simulink model "RobotArmControl"  (R2014a)
settings: Solver=ode45  StartTime=0.0  StopTime=10  RelTol=1e-3
values from neighbouring files (symbols this model uses):
  a1 = 0    [MainRobotControl.m]    (also in RobotParameters.m; Trajectory_PlanningRot.m; Trajectory_planning.m = x0; taskspace_v1.m = 5.66666666667)
  a2 = 0.2    [MainRobotControl.m]    (also in RobotParameters.m; Trajectory_PlanningRot.m = 0; Trajectory_planning.m = xdot0; taskspace_v1.m = 20)
  a3 = 0.2    [MainRobotControl.m]    (also in RobotParameters.m; Trajectory_PlanningRot.m = (3*h - (2*thetadot_0 + thetadot_f)*T)/(T*T); Trajectory_planning.m = (3*h - (2*xdot0 + xdotf)*T)/(T*T); taskspace_v1.m = 26.8333333333)
  d1 = 0.2    [MainRobotControl.m]    (also in RobotParameters.m; taskspace_v1.m = 15.8333333333)
  d5 = 0.07    [MainRobotControl.m]    (also in RobotParameters.m; taskspace_v1.m = 10)
  gear_eff = 0.85    [RobotParameters.m]
  kphi = 37.83e-3    (= 0.03783)    [RobotParameters.m]
  Kv = 4.09e-4    (= 0.000409)    [RobotParameters.m]
  Ra = 5.84    [RobotParameters.m]
  ratio = 19    [RobotParameters.m]
  tau_e = La/Ra    (= 9.58904109589e-05)    [RobotParameters.m]
  tau_m = Jrob/Kv    (= 8.25476772616)    [RobotParameters.m]
libraries: simulink x6
settings Model: Creator=Guillaume  LastModifiedBy=Guillaume

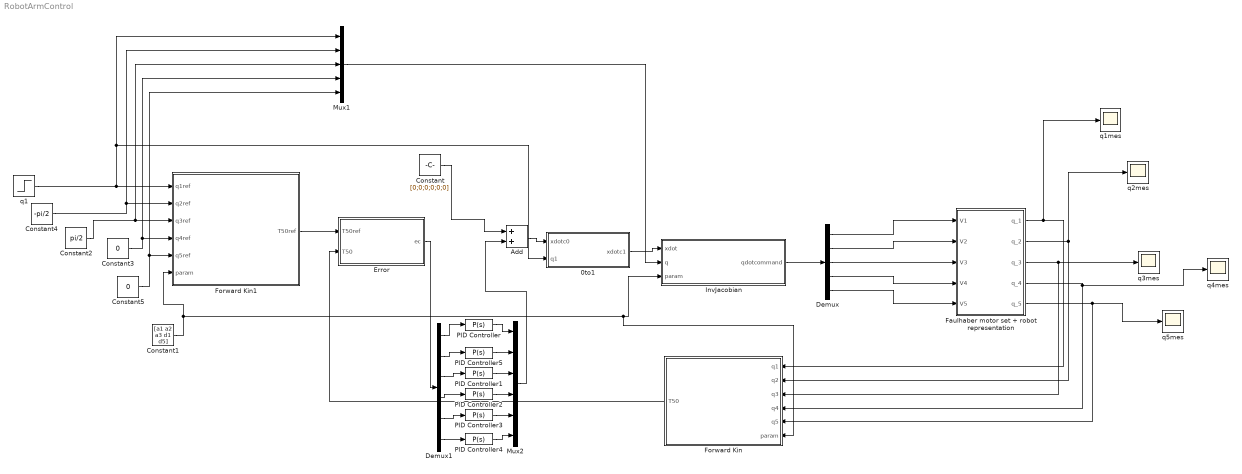
== system RobotArmControl ==
  0to1 : MATLAB Function  TreatAsAtomicUnit=on
  Add : Sum
  Constant : Constant  Value=[0;0;0;0;0;0]
  Constant1 : Constant  Value=[a1 a2 a3 d1 d5]
  Constant2 : Constant  Value=pi/2
  Constant3 : Constant  Value=0
  Constant4 : Constant  Value=-pi/2
  Constant5 : Constant  Value=0
  Demux : Demux  Outputs=5
  Demux1 : Demux  Outputs=6
  Error : MATLAB Function  TreatAsAtomicUnit=on
  Faulhaber motor set + robot representation : Subsystem
  Forward Kin : MATLAB Function  TreatAsAtomicUnit=on
  Forward Kin1 : MATLAB Function  TreatAsAtomicUnit=on
  InvJacobian : MATLAB Function  TreatAsAtomicUnit=on
  Mux1 : Mux  Inputs=5
  Mux2 : Mux  Inputs=6
  PID Controller{,1..5} (6 alike) : simulink/Continuous/PID Controller  Controller=P  TimeDomain=Continuous-time  SampleTime=1  IntegratorMethod=Forward Euler  FilterMethod=Forward Euler  Form=Parallel  P=1e-5  I=1  D=0  N=100  InitialConditionSource=internal  InitialConditionForIntegrator=0  InitialConditionForFilter=0  ExternalReset=none  LimitOutput=off  UpperSaturationLimit=inf  LowerSaturationLimit=-inf  LinearizeAsGain=on  AntiWindupMode=none  Kb=1  TrackingMode=off  Kt=1  PParamMin=[]  PParamMax=[]  IParamMin=[]  IParamMax=[]  DParamMin=[]  DParamMax=[]  NParamMin=[]  NParamMax=[]  KbParamMin=[]  KbParamMax=[]  KtParamMin=[]  KtParamMax=[]  POutMin=[]  POutMax=[]  IOutMin=[]  IOutMax=[]  DOutMin=[]  DOutMax=[]  NOutMin=[]  NOutMax=[]  KbOutMin=[]  KbOutMax=[]  KtOutMin=[]  KtOutMax=[]  IntegratorOutMin=[]  IntegratorOutMax=[]  FilterOutMin=[]  FilterOutMax=[]  SumOutMin=[]  SumOutMax=[]  SumI1OutMin=[]  SumI1OutMax=[]  SumI2OutMin=[]  SumI2OutMax=[]  SumI3OutMin=[]  SumI3OutMax=[]  SumDOutMin=[]  SumDOutMax=[]  SaturationOutMin=[]  SaturationOutMax=[]  IntegratorContinuousStateAttributes=''  IntegratorStateMustResolveToSignalObject=off  IntegratorRTWStateStorageClass=Auto  FilterContinuousStateAttributes=''  FilterStateMustResolveToSignalObject=off  FilterRTWStateStorageClass=Auto
  q1 : Step  After=pi/20  SampleTime=0
  q1mes : Scope
  q2mes : Scope
  q3mes : Scope
      settings: SaveName=ScopeData2
  q4mes : Scope
      settings: SaveName=ScopeData3
  q5mes : Scope
      settings: SaveName=ScopeData4
  wires:
  Faulhaber motor set + robot representation/1(q_1) -> q1mes/1, Forward Kin/1(q1)
  Faulhaber motor set + robot representation/2(q_2) -> Forward Kin/2(q2), q2mes/1
  Faulhaber motor set + robot representation/3(q_3) -> q3mes/1, Forward Kin/3(q3)
  Faulhaber motor set + robot representation/4(q_4) -> q4mes/1, Forward Kin/4(q4)
  Faulhaber motor set + robot representation/5(q_5) -> q5mes/1, Forward Kin/5(q5)
  InvJacobian/1(qdotcommand) -> Demux/1
  Demux/1 -> Faulhaber motor set + robot representation/1(V1)
  Demux/2 -> Faulhaber motor set + robot representation/2(V2)
  Demux/3 -> Faulhaber motor set + robot representation/3(V3)
  Demux/4 -> Faulhaber motor set + robot representation/4(V4)
  Demux/5 -> Faulhaber motor set + robot representation/5(V5)
  0to1/1(xdotc1) -> InvJacobian/1(xdot)
  Add/1 -> 0to1/1(xdotc0)
  Constant/1 -> Add/1
  Forward Kin/1(T50) -> Error/2(T50)
  Forward Kin1/1(T50ref) -> Error/1(T50ref)
  q1/1 -> 0to1/2(q1), Mux1/1, Forward Kin1/1(q1ref)
  Constant4/1 -> Mux1/2, Forward Kin1/2(q2ref)
  Constant2/1 -> Mux1/3, Forward Kin1/3(q3ref)
  Constant3/1 -> Mux1/4, Forward Kin1/4(q4ref)
  Constant5/1 -> Mux1/5, Forward Kin1/5(q5ref)
  Mux1/1 -> InvJacobian/2(q)
  Constant1/1 -> Forward Kin/6(param), InvJacobian/3(param), Forward Kin1/6(param)
  Error/1(ec) -> Demux1/1
  Demux1/1 -> PID Controller/1
  PID Controller/1 -> Mux2/1
  PID Controller4/1 -> Mux2/6
  Demux1/6 -> PID Controller4/1
  Demux1/5 -> PID Controller3/1
  PID Controller3/1 -> Mux2/5
  Demux1/4 -> PID Controller2/1
  PID Controller2/1 -> Mux2/4
  Demux1/3 -> PID Controller1/1
  PID Controller1/1 -> Mux2/3
  PID Controller5/1 -> Mux2/2
  Demux1/2 -> PID Controller5/1
  Mux2/1 -> Add/2

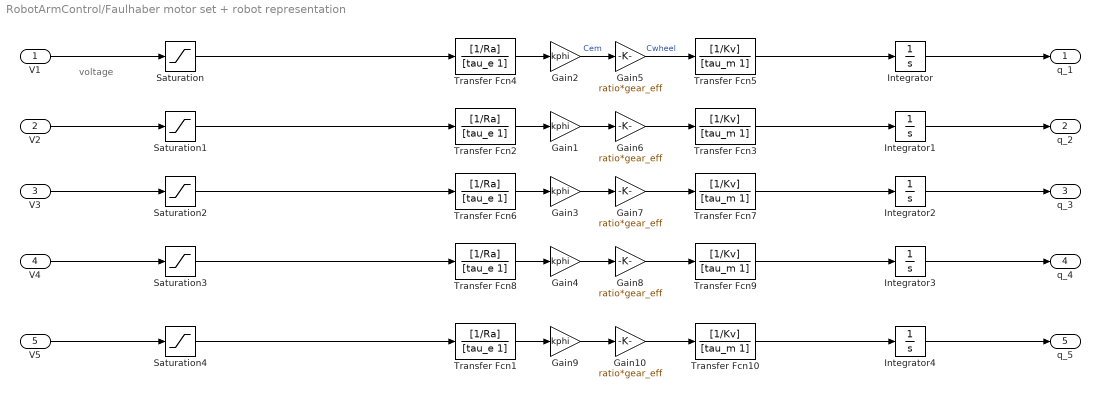
== system RobotArmControl/Faulhaber motor set + robot representation ==
  note: voltage
  V1 : Inport
  V2 : Inport  Port=2
  V3 : Inport  Port=3
  V4 : Inport  Port=4
  V5 : Inport  Port=5
  Gain{1..4,9} (5 alike) : Gain  Gain=kphi
  Gain{5..8,10} (5 alike) : Gain  Gain=ratio*gear_eff
  Integrator{,1..4} (5 alike) : Integrator
  Saturation{,1..4} (5 alike) : Saturate  UpperLimit=52/0.036
  Transfer Fcn{1..2,4,6,8} (5 alike) : TransferFcn  Numerator=[1/Ra]  Denominator=[tau_e 1]
  Transfer Fcn{3,5,7,9..10} (5 alike) : TransferFcn  Numerator=[1/Kv]  Denominator=[tau_m 1]
  q_1 : Outport
  q_2 : Outport  Port=2
  q_3 : Outport  Port=3
  q_4 : Outport  Port=4
  q_5 : Outport  Port=5
  wires:
  Transfer Fcn5/1 -> Integrator/1
  Saturation/1 -> Transfer Fcn4/1
  Transfer Fcn3/1 -> Integrator1/1
  V2/1 -> Saturation1/1
  Saturation1/1 -> Transfer Fcn2/1
  V1/1 -> Saturation/1
  Transfer Fcn7/1 -> Integrator2/1
  V3/1 -> Saturation2/1
  Saturation2/1 -> Transfer Fcn6/1
  Transfer Fcn9/1 -> Integrator3/1
  V4/1 -> Saturation3/1
  Saturation3/1 -> Transfer Fcn8/1
  Transfer Fcn2/1 -> Gain1/1
  Gain1/1 -> Gain6/1
  Transfer Fcn4/1 -> Gain2/1
  Gain2/1 -> Gain5/1  "Cem"
  Transfer Fcn6/1 -> Gain3/1
  Gain3/1 -> Gain7/1
  Transfer Fcn8/1 -> Gain4/1
  Gain4/1 -> Gain8/1
  Gain5/1 -> Transfer Fcn5/1  "Cwheel"
  Gain6/1 -> Transfer Fcn3/1
  Gain7/1 -> Transfer Fcn7/1
  Gain8/1 -> Transfer Fcn9/1
  Integrator/1 -> q_1/1
  Integrator3/1 -> q_4/1
  Integrator2/1 -> q_3/1
  Integrator1/1 -> q_2/1
  Transfer Fcn10/1 -> Integrator4/1
  V5/1 -> Saturation4/1
  Saturation4/1 -> Transfer Fcn1/1
  Transfer Fcn1/1 -> Gain9/1
  Gain9/1 -> Gain10/1
  Gain10/1 -> Transfer Fcn10/1
  Integrator4/1 -> q_5/1

== matlab function RobotArmControl/InvJacobian ==
  data: xdot input; qdotcommand output; q input; param input
function qdotcommand   = InvJacobian5by5(xdot,q,param)
%UNTITLED2 Summary of this function goes here
%   Detailed explanation goes here

%ATTENTION xdot must be expressed in referential 1 !!
%note  : pas de prise en compte d'une commande de omega sur x1.
%supposée zero tout le temps

% invJ5by5 = [                                                                                        0,                                                                                        0,                     1/(a1 + a3*cos(t2 + t3) + a2*cos(t2) - d5*sin(t2 + t3 + t4)),                   0,                                                                                                                                                                                                           0;
%                         -cos(t2 + t3)/(a2*cos(t2 + t3)*sin(t2) - a2*sin(t2 + t3)*cos(t2)),                        -sin(t2 + t3)/(a2*cos(t2 + t3)*sin(t2) - a2*sin(t2 + t3)*cos(t2)),                                                                                0,                   0,                                                                                -(d5*cos(t2 + t3 + t4)*cos(t2 + t3) + d5*sin(t2 + t3 + t4)*sin(t2 + t3))/(a2*cos(t2 + t3)*sin(t2) - a2*sin(t2 + t3)*cos(t2));
%  (a3*cos(t2 + t3) + a2*cos(t2))/(a2*a3*cos(t2 + t3)*sin(t2) - a2*a3*sin(t2 + t3)*cos(t2)), (a3*sin(t2 + t3) + a2*sin(t2))/(a2*a3*cos(t2 + t3)*sin(t2) - a2*a3*sin(t2 + t3)*cos(t2)),                                                                                0,                   0, (a3*d5*sin(t2 + t3 + t4)*sin(t2 + t3) + a2*d5*cos(t2 + t3 + t4)*cos(t2) + a2*d5*sin(t2 + t3 + t4)*sin(t2) + a3*d5*cos(t2 + t3 + t4)*cos(t2 + t3))/(a2*a3*cos(t2 + t3)*sin(t2) - a2*a3*sin(t2 + t3)*cos(t2));
%                              -cos(t2)/(a3*cos(t2 + t3)*sin(t2) - a3*sin(t2 + t3)*cos(t2)),                             -sin(t2)/(a3*cos(t2 + t3)*sin(t2) - a3*sin(t2 + t3)*cos(t2)),                                                                                0,                   0,                                      -(a3*sin(t2 + t3)*cos(t2) - a3*cos(t2 + t3)*sin(t2) + d5*cos(t2 + t3 + t4)*cos(t2) + d5*sin(t2 + t3 + t4)*sin(t2))/(a3*cos(t2 + t3)*sin(t2) - a3*sin(t2 + t3)*cos(t2));
%                                                                                         0,                                                                                        0, 1/(cos(t2 + t3 + t4)*(a1 + a3*cos(t2 + t3) + a2*cos(t2) - d5*sin(t2 + t3 + t4))), 1/cos(t2 + t3 + t4),                                                                                                                                                                                                           0];

a1 = param(1);
a2 = param(2);
a3 = param(3);
%d1 = param(4);
d5 = param(5);

%t1 = q(1);
t2 = q(2);
t3 = q(3);
t4 = q(4);
%t5 = q(5);


invJ5by5 = [                                    0,                                               0,                     1/(a1 + a3*cos(t2 + t3) + a2*cos(t2) - d5*sin(t2 + t3 + t4)),                   0,                                                    0;
                       cos(t2 + t3)/(a2*sin(t3)),                       sin(t2 + t3)/(a2*sin(t3)),                                                                                0,                   0,                            (d5*cos(t4))/(a2*sin(t3));
 -(a3*cos(t2 + t3) + a2*cos(t2))/(a2*a3*sin(t3)), -(a3*sin(t2 + t3) + a2*sin(t2))/(a2*a3*sin(t3)),                                                                                0,                   0, -(d5*(a2*cos(t3 + t4) + a3*cos(t4)))/(a2*a3*sin(t3));
                            cos(t2)/(a3*sin(t3)),                            sin(t2)/(a3*sin(t3)),                                                                                0,                   0,          (d5*cos(t3 + t4) + a3*sin(t3))/(a3*sin(t3));
                                               0,                                               0, 1/(cos(t2 + t3 + t4)*(a1 + a3*cos(t2 + t3) + a2*cos(t2) - d5*sin(t2 + t3 + t4))), 1/cos(t2 + t3 + t4),                                                    0];
indice = [1 2 3 5 6];                                                                                   



qdotcommand = invJ5by5*xdot(indice);
                                           
end

== matlab function RobotArmControl/Forward Kin ==
  data: q1 input; T50 output; q2 input; q3 input; q4 input; q5 input; param input
function T50 = FK(q1,q2,q3,q4,q5,param)
%#codegen

a1 = param(1);
a2 = param(2);
a3 = param(3);
d1 = param(4);
d5 = param(5);

t1 = q1;
t2 = q2;
t3 = q3;
t4 = q4;
t5 = q5;

T50 = zeros(4,4);

T50 = [ sin(t1)*sin(t5) + cos(t2 + t3 + t4)*cos(t1)*cos(t5),   cos(t5)*sin(t1) - cos(t2 + t3 + t4)*cos(t1)*sin(t5), -sin(t2 + t3 + t4)*cos(t1), cos(t1)*(a1 + a3*cos(t2 + t3) + a2*cos(t2) - d5*sin(t2 + t3 + t4));
        cos(t2 + t3 + t4)*cos(t5)*sin(t1) - cos(t1)*sin(t5), - cos(t1)*cos(t5) - cos(t2 + t3 + t4)*sin(t1)*sin(t5), -sin(t2 + t3 + t4)*sin(t1), sin(t1)*(a1 + a3*cos(t2 + t3) + a2*cos(t2) - d5*sin(t2 + t3 + t4));
                                 -sin(t2 + t3 + t4)*cos(t5),                             sin(t2 + t3 + t4)*sin(t5),         -cos(t2 + t3 + t4),           d1 - a3*sin(t2 + t3) - a2*sin(t2) - d5*cos(t2 + t3 + t4);
                                                          0,                                                     0,                          0,                                                                  1];

== matlab function RobotArmControl/0to1 ==
  data: xdotc0 input; xdotc1 output; q1 input
function xdotc1 = RotationMatrix(xdotc0,q1)
%#codegen

t1 = q1;

R01 = [  cos(t1), sin(t1),  0;
        0,       0, -1;
 -sin(t1), cos(t1),  0];

xdotc1 = zeros(6,1);

xdotc1(1:3) = R01*xdotc0(1:3);
xdotc1(4:6) = R01*xdotc0(4:6);

== matlab function RobotArmControl/Error ==
  data: T50ref input; ec output; T50 input
function ec  = Compute_error(T50ref,T50)
%UNTITLED Summary of this function goes here
%   Detailed explanation goes here

x = T50(1:3,4);
R = T50(1:3,1:3);

xref = T50ref(1:3,4);
Rref = T50ref(1:3,1:3);

etr = xref - x;

eor = (1/2)*(cross(R(:,1),Rref(:,1)) + cross(R(:,2),Rref(:,2)) + cross(R(:,3),Rref(:,3)));

ec = [etr;eor];


end

== matlab function RobotArmControl/Forward Kin1 ==
  data: q1ref input; T50ref output; q2ref input; q3ref input; q4ref input; q5ref input; param input
function T50ref = FKref(q1ref,q2ref,q3ref,q4ref,q5ref,param)
%#codegen

a1 = param(1);
a2 = param(2);
a3 = param(3);
d1 = param(4);
d5 = param(5);

t1 = q1ref;
t2 = q2ref;
t3 = q3ref;
t4 = q4ref;
t5 = q5ref;

T50ref = [ sin(t1)*sin(t5) + cos(t2 + t3 + t4)*cos(t1)*cos(t5),   cos(t5)*sin(t1) - cos(t2 + t3 + t4)*cos(t1)*sin(t5), -sin(t2 + t3 + t4)*cos(t1), cos(t1)*(a1 + a3*cos(t2 + t3) + a2*cos(t2) - d5*sin(t2 + t3 + t4));
        cos(t2 + t3 + t4)*cos(t5)*sin(t1) - cos(t1)*sin(t5), - cos(t1)*cos(t5) - cos(t2 + t3 + t4)*sin(t1)*sin(t5), -sin(t2 + t3 + t4)*sin(t1), sin(t1)*(a1 + a3*cos(t2 + t3) + a2*cos(t2) - d5*sin(t2 + t3 + t4));
                                 -sin(t2 + t3 + t4)*cos(t5),                             sin(t2 + t3 + t4)*sin(t5),         -cos(t2 + t3 + t4),           d1 - a3*sin(t2 + t3) - a2*sin(t2) - d5*cos(t2 + t3 + t4);
                                                          0,                                                     0,                          0,                                                                  1];
